simulink model "TrainingTracerVer3"  (R2025b)
settings: Solver=FixedStepAuto  StartTime=0.0  StopTime=inf  RelTol=1e-3  EnableMultiTasking=on
undefined symbols (not defined in the file): bits
libraries: stm32blockslib x11, stm32f4xxblockslib x10, svdutilitieslib x6
settings Model: STM32="{\"DigitalPortWrite\":[{\"ID\":\"Tracer_New_Version:271\"},{\"ID\":\"Tracer_New_Version:279\"},{\"ID\":\"Tracer_New_Version:277\"},{\"ID\":\"Tracer_New_Version:262\"},{\"ID\":\"TrainingTracerVer3:279\"},{\"ID\":\"TrainingTracerVer3:277\"},{\"ID\":\"TrainingTracerVer3:262\"},{\"ID\":\"TrainingTracerVer3:271\"}],\"EncoderBlock\":[{\"ID\":\"Tracer_New_Version:4\"},{\"ID\":\"Tracer_New_Version:3\"},{\"ID\":\"TrainingTracerVer3:4\"},{\"ID\":\"TrainingTracerVer3:3\"}],\"PWMOutput\":[{\"ID\":\"Tracer_New_Version:280\"},{\"ID\":\"Tracer_New_Version:278\"},{\"ID\":\"TrainingTracerVer3:280\"},{\"ID\":\"TrainingTracerVer3:278\"}],\"AnalogInput\":[{\"ID\":\"Tracer_New_Version:227\"},{\"ID\":\"Tracer_New_Version:226\"},{\"ID\":\"TrainingTracerVer3:226\"},{\"ID\":\"TrainingTracerVer3:227\"}],\"I2CControllerRead\":[{\"ID\":\"Tracer_New_Version:61\"},{\"ID\":\"Tracer_New_Version:124\"},{\"ID\":\"Tracer_New_Version:123\"},{\"ID\":\"Tracer_New_Version:187\"},{\"ID\":\"Tracer_New_Version:186\"},{\"ID\":\"Tracer_New_Version:81\"},{\"ID\":\"Tracer_New_Version:80\"},{\"ID\":\"Tracer_New_Version:144\"},{\"ID\":\"Tracer_New_Version:143\"},{\"ID\":\"Tracer_New_Version:207\"},{\"ID\":\"Tracer_New_Version:206\"},{\"ID\":\"Tracer_New_Version:103\"},{\"ID\":\"Tracer_New_Version:102\"},{\"ID\":\"Tracer_New_Version:166\"},{\"ID\":\"Tracer_New_Version:165\"},{\"ID\":\"TrainingTracerVer3:61\"},{\"ID\":\"TrainingTracerVer3:81\"},{\"ID\":\"TrainingTracerVer3:124\"},{\"ID\":\"TrainingTracerVer3:144\"},{\"ID\":\"TrainingTracerVer3:187\"},{\"ID\":\"TrainingTracerVer3:207\"}],\"DigitalPortRead\":[{\"ID\":\"Tracer_New_Version:237\"},{\"ID\":\"Tracer_New_Version:236\"},{\"ID\":\"TrainingTracerVer3:236\"},{\"ID\":\"TrainingTracerVer3:237\"}],\"I2CControllerWrite\":[{\"ID\":\"Tracer_New_Version:41\"},{\"ID\":\"Tracer_New_Version:42\"},{\"ID\":\"Tracer_New_Version:43\"},{\"ID\":\"TrainingTracerVer3:41\"},{\"ID\":\"TrainingTracerVer3:42\"},{\"ID\":\"TrainingTracerVer3:43\"}]}"  Creator=niijima  LastModifiedBy=niijima
settings OptimizationCC: EnhancedBackFolding=on  PassReuseOutputArgsAs=Individual arguments  ZeroExternalMemoryAtStartup=off  ZeroInternalMemoryAtStartup=off  MaxStackSize=512  OptimizeBlockOrder=speed  DifferentSizesBufferReuse=on  OptimizationCustomize=off  EfficientTunableParamExpr=on
settings DebuggingCC: ParameterTunabilityLossMsg=error
settings HardwareCC: ProdBitPerPointer=32.0  ProdBitPerSizeT=32.0  ProdBitPerPtrDiffT=32.0  ProdLargestAtomicInteger=Long  ProdLargestAtomicFloat=Double  ProdWordSize=32.0  ProdLongLongMode=on  ProdHWDeviceType=ARM Compatible->ARM Cortex-M
settings SFSimCC: MATLABDynamicMemAlloc=off
settings RTWCC: SystemTargetFile=ert.tlc  HardwareBoard=STM32F3xx Based  TemplateMakefile=ert_default_tmf  Toolchain=GNU Tools for ARM Embedded Processors  BuildConfiguration=Faster Runs  Description=Embedded Coder
settings CodeAppCC: ForceParamTrailComments=on  IgnoreCustomStorageClasses=off  OperatorAnnotations=on  SimulinkDataObjDesc=on  SFDataObjDesc=on  InsertBlockDesc=on
settings ERTTargetCC: ExtModeTransport=3.0  ExtModeStaticAlloc=on  ExtModeStaticAllocSize=2048.0  ExtModeMexFile=ext_xcp  ExtModeIntrfLevel=Level2 - Open  InlinedParameterPlacement=Hierarchical  DynamicArrayContainerType=coder::array  TargetLangStandard=C99 (ISO)  CodeReplacementLibrary=ARM Cortex-M  SupportContinuousTime=on

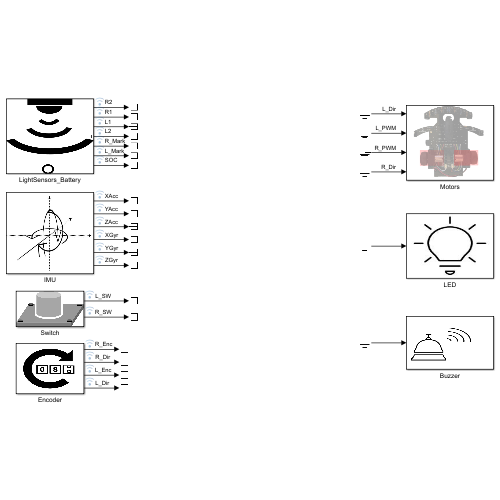
[thumbnail: Simulink's stored preview of the top-level diagram]
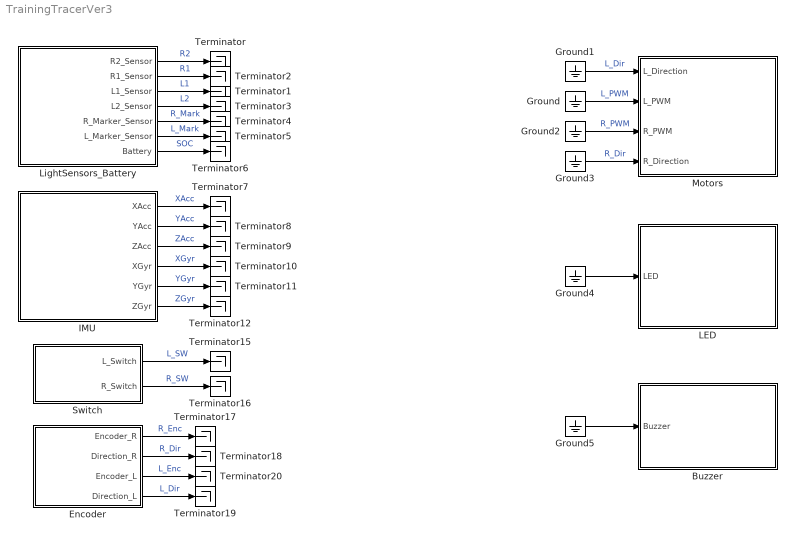
== system TrainingTracerVer3 ==
  Buzzer : Subsystem
      mask Display: image('Picture2.png');
  Encoder : Subsystem
      mask Display: image('c1d4fd0d-d243-4f64-b1ab-5e56abbdef7e.jpg');
  Ground{,1..5} (6 alike) : Ground
  IMU : Subsystem
      mask Display: image('55213469-1105-4cd9-b002-0902cf504a17.jpg');
  LED : Subsystem
      mask Display: image('c54385e9-ac3c-4890-af1e-d5685341beff.jpg');
  LightSensors_Battery : Subsystem
      mask Display: image('6109ffca-7121-49e0-b053-0876b8c7f2a6.jpg');
  Motors : Subsystem
      mask Display: image('Picture1.png');
  Switch : Subsystem
      mask Display: image('画像 (2).png');
  Terminator{,1..12,15..20} (19 alike) : Terminator
  wires:
  Encoder/2(Direction_R) -> Terminator18/1  "R_Dir"
  Encoder/1(Encoder_R) -> Terminator17/1  "R_Enc"
  Switch/2(R_Switch) -> Terminator16/1  "R_SW"
  Switch/1(L_Switch) -> Terminator15/1  "L_SW"
  IMU/6(ZGyr) -> Terminator12/1  "ZGyr"
  IMU/5(YGyr) -> Terminator11/1  "YGyr"
  IMU/4(XGyr) -> Terminator10/1  "XGyr"
  IMU/3(ZAcc) -> Terminator9/1  "ZAcc"
  IMU/2(YAcc) -> Terminator8/1  "YAcc"
  IMU/1(XAcc) -> Terminator7/1  "XAcc"
  LightSensors_Battery/7(Battery) -> Terminator6/1  "SOC"
  LightSensors_Battery/6(L_Marker_Sensor) -> Terminator5/1  "L_Mark"
  LightSensors_Battery/5(R_Marker_Sensor) -> Terminator4/1  "R_Mark"
  LightSensors_Battery/4(L2_Sensor) -> Terminator3/1  "L2"
  LightSensors_Battery/3(L1_Sensor) -> Terminator1/1  "L1"
  LightSensors_Battery/2(R1_Sensor) -> Terminator2/1  "R1"
  LightSensors_Battery/1(R2_Sensor) -> Terminator/1  "R2"
  Ground/1 -> Motors/2(L_PWM)  "L_PWM"
  Ground5/1 -> Buzzer/1(Buzzer)
  Ground4/1 -> LED/1(LED)
  Ground2/1 -> Motors/3(R_PWM)  "R_PWM"
  Ground1/1 -> Motors/1(L_Direction)  "L_Dir"
  Encoder/4(Direction_L) -> Terminator19/1  "L_Dir"
  Encoder/3(Encoder_L) -> Terminator20/1  "L_Enc"
  Ground3/1 -> Motors/4(R_Direction)  "R_Dir"

== system TrainingTracerVer3/Buzzer ==
  Buzzer : Inport
  Buzzer_ : stm32f4xxblockslib/Digital Port Write  PortName=GPIOA  PinNumber=[12]  ReadOperation=off  IOAsArray=on  EnableSimPort=off  hoistedMaskSrc=ECSoC/ECSimCodegen/Digital Port Write
      settings: LibrarySourceBlock=stm32f3xxblockslib/Digital Port Write
  wires:
  Buzzer/1 -> Buzzer_/1

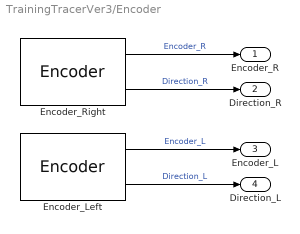
== system TrainingTracerVer3/Encoder ==
  Encoder_Left : stm32blockslib/Encoder  TimerModule=TIM1  EnableResetInput=off  OutputDirection=on  SampleTime=-1
      settings: LibrarySourceBlock=stm32f3xxblockslib/Encoder
  Encoder_Right : stm32blockslib/Encoder  TimerModule=TIM2  EnableResetInput=off  OutputDirection=on  SampleTime=-1
      settings: LibrarySourceBlock=stm32f3xxblockslib/Encoder
  Encoder_R : Outport
  Direction_R : Outport  Port=2
  Encoder_L : Outport  Port=3
  Direction_L : Outport  Port=4
  wires:
  Encoder_Right/2 -> Direction_R/1  "Direction_R"
  Encoder_Right/1 -> Encoder_R/1  "Encoder_R"
  Encoder_Left/1 -> Encoder_L/1  "Encoder_L"
  Encoder_Left/2 -> Direction_L/1  "Direction_L"

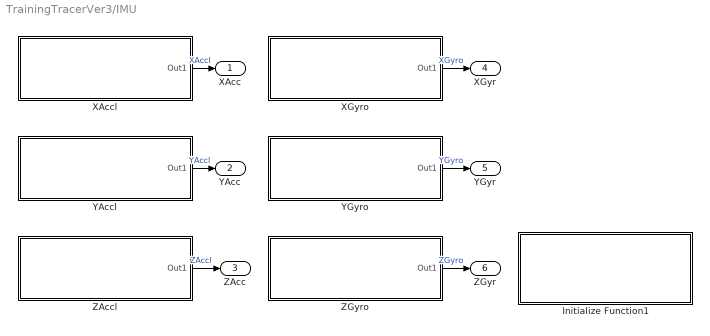
== system TrainingTracerVer3/IMU ==
  Initialize Function1 : Subsystem  TreatAsAtomicUnit=on
  XAccl : Subsystem
  XGyro : Subsystem
  YAccl : Subsystem
  YGyro : Subsystem
  ZAccl : Subsystem
  ZGyro : Subsystem
  XAcc : Outport
  YAcc : Outport  Port=2
  ZAcc : Outport  Port=3
  XGyr : Outport  Port=4
  YGyr : Outport  Port=5
  ZGyr : Outport  Port=6
  wires:
  YGyro/1(Out1) -> YGyr/1  "YGyro"
  ZGyro/1(Out1) -> ZGyr/1  "ZGyro"
  ZAccl/1(Out1) -> ZAcc/1  "ZAccl"
  XGyro/1(Out1) -> XGyr/1  "XGyro"
  YAccl/1(Out1) -> YAcc/1  "YAccl"
  XAccl/1(Out1) -> XAcc/1  "XAccl"

== system TrainingTracerVer3/LED ==
  LED : Inport
  LED_ : stm32f4xxblockslib/Digital Port Write  PortName=GPIOB  PinNumber=[3]  ReadOperation=off  IOAsArray=on  EnableSimPort=off  hoistedMaskSrc=ECSoC/ECSimCodegen/Digital Port Write
      settings: LibrarySourceBlock=stm32f3xxblockslib/Digital Port Write
  wires:
  LED/1 -> LED_/1

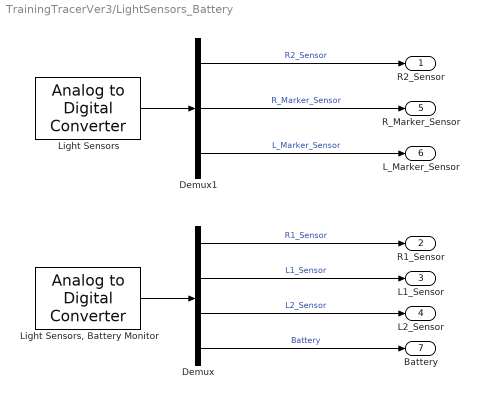
== system TrainingTracerVer3/LightSensors_Battery ==
  Demux : Demux
  Demux1 : Demux  Outputs=3
  Light Sensors : stm32f4xxblockslib/Analog to Digital Converter  ADCModule=ADC1  ConversionGroup=Regular  TriggerMode=Trigger and read  NumberOfConversions=3  EnableBufferConv=off  BufferLength=1  OutputStatus=off  SampleTime=-1  EnableSimPort=off  hoistedMaskSrc=ECSoC/ECSimCodegen/Analog to Digital Converter
      settings: LibrarySourceBlock=stm32f3xxblockslib/Analog to Digital Converter
  "Light Sensors, Battery Monitor" : stm32f4xxblockslib/Analog to Digital Converter  ADCModule=ADC2  ConversionGroup=Regular  TriggerMode=Trigger and read  NumberOfConversions=4  EnableBufferConv=off  BufferLength=1  OutputStatus=off  SampleTime=-1  EnableSimPort=off  hoistedMaskSrc=ECSoC/ECSimCodegen/Analog to Digital Converter
      settings: LibrarySourceBlock=stm32f3xxblockslib/Analog to Digital Converter
  R2_Sensor : Outport
  R1_Sensor : Outport  Port=2
  L1_Sensor : Outport  Port=3
  L2_Sensor : Outport  Port=4
  R_Marker_Sensor : Outport  Port=5
  L_Marker_Sensor : Outport  Port=6
  Battery : Outport  Port=7
  wires:
  Demux/2 -> L1_Sensor/1  "L1_Sensor"
  "Light Sensors, Battery Monitor"/1 -> Demux/1
  Demux1/1 -> R2_Sensor/1  "R2_Sensor"
  Light Sensors/1 -> Demux1/1
  Demux/3 -> L2_Sensor/1  "L2_Sensor"
  Demux1/3 -> L_Marker_Sensor/1  "L_Marker_Sensor"
  Demux1/2 -> R_Marker_Sensor/1  "R_Marker_Sensor"
  Demux/4 -> Battery/1  "Battery"
  Demux/1 -> R1_Sensor/1  "R1_Sensor"

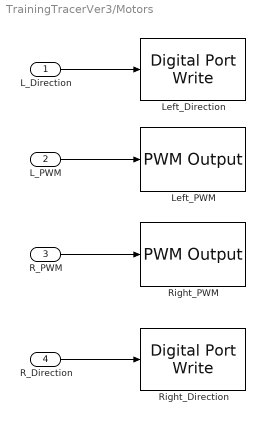
== system TrainingTracerVer3/Motors ==
  L_Direction : Inport
  L_PWM : Inport  Port=2
  R_PWM : Inport  Port=3
  R_Direction : Inport  Port=4
  Left_Direction : stm32f4xxblockslib/Digital Port Write  PortName=GPIOA  PinNumber=[10]  ReadOperation=off  IOAsArray=on  EnableSimPort=off  hoistedMaskSrc=ECSoC/ECSimCodegen/Digital Port Write
      settings: LibrarySourceBlock=stm32f3xxblockslib/Digital Port Write
  Left_PWM : stm32f4xxblockslib/PWM Output  ProcessorFamily=STM32F3  TimerModule=TIM16  DutycycleUnits=Percentage  EnableChannel1=on  EnableCaptureCompare1Input=off  EnableCaptureCompare1ComplementaryInput=off  EnableOutputCompare1ModeInput=off  EnableChannel2=off  EnableCaptureCompare2Input=off  EnableCaptureCompare2ComplementaryInput=off  EnableOutputCompare2ModeInput=off  EnableChannel3=off  EnableCaptureCompare3Input=off  EnableCaptureCompare3ComplementaryInput=off  EnableOutputCompare3ModeInput=off  EnableChannel4=on  EnableCaptureCompare4Input=off  EnableCaptureCompare4ComplementaryInput=off  EnableOutputCompare4ModeInput=off  EnableChannel5=off  EnableCaptureCompare5Input=off  EnableOutputCompare5ModeInput=off  EnableChannel6=off  EnableCaptureCompare6Input=off  EnableOutputCompare6ModeInput=off  EnableCounterInput=off  EnableMainOutputInput=off  EnableFrequencyInput=off  SetRCAfterCE=off  OutputDirection=off  OutputMainOutputEnableStatus=off  SampleTime=0.1  EnableSimPort=off  EnableUpdateEvent=off  EnableCaptureCompare1Event=off  EnableCaptureCompare2Event=off  EnableCaptureCompare3Event=off  EnableCaptureCompare4Event=off  EnableTriggerEvent=off  EnableBreakEvent=off  EnableBreakEvent2=off  hoistedMaskSrc=ECSoC/ECSimCodegen/PWM Output
      settings: LibrarySourceBlock=stm32f3xxblockslib/PWM Output
  Right_Direction : stm32f4xxblockslib/Digital Port Write  PortName=GPIOA  PinNumber=[11]  ReadOperation=off  IOAsArray=on  EnableSimPort=off  hoistedMaskSrc=ECSoC/ECSimCodegen/Digital Port Write
      settings: LibrarySourceBlock=stm32f3xxblockslib/Digital Port Write
  Right_PWM : stm32f4xxblockslib/PWM Output  ProcessorFamily=STM32F3  TimerModule=TIM17  DutycycleUnits=Percentage  EnableChannel1=on  EnableCaptureCompare1Input=off  EnableCaptureCompare1ComplementaryInput=off  EnableOutputCompare1ModeInput=off  EnableChannel2=off  EnableCaptureCompare2Input=off  EnableCaptureCompare2ComplementaryInput=off  EnableOutputCompare2ModeInput=off  EnableChannel3=off  EnableCaptureCompare3Input=off  EnableCaptureCompare3ComplementaryInput=off  EnableOutputCompare3ModeInput=off  EnableChannel4=off  EnableCaptureCompare4Input=off  EnableCaptureCompare4ComplementaryInput=off  EnableOutputCompare4ModeInput=off  EnableChannel5=off  EnableCaptureCompare5Input=off  EnableOutputCompare5ModeInput=off  EnableChannel6=off  EnableCaptureCompare6Input=off  EnableOutputCompare6ModeInput=off  EnableCounterInput=off  EnableMainOutputInput=off  EnableFrequencyInput=off  SetRCAfterCE=off  OutputDirection=off  OutputMainOutputEnableStatus=off  SampleTime=0.1  EnableSimPort=off  EnableUpdateEvent=off  EnableCaptureCompare1Event=off  EnableCaptureCompare2Event=off  EnableCaptureCompare3Event=off  EnableCaptureCompare4Event=off  EnableTriggerEvent=off  EnableBreakEvent=off  EnableBreakEvent2=off  hoistedMaskSrc=ECSoC/ECSimCodegen/PWM Output
      settings: LibrarySourceBlock=stm32f3xxblockslib/PWM Output
  wires:
  R_Direction/1 -> Right_Direction/1
  R_PWM/1 -> Right_PWM/1
  L_Direction/1 -> Left_Direction/1
  L_PWM/1 -> Left_PWM/1

== system TrainingTracerVer3/Switch ==
  L_Switch_ : stm32f4xxblockslib/Digital Port Read  PortName=GPIOF  PinNumber=[0]  ReadOperation=on  IOAsArray=off  SampleTime=-1  EnableSimPort=off  hoistedMaskSrc=ECSoC/ECSimCodegen/Digital Port Read
      settings: LibrarySourceBlock=stm32f3xxblockslib/Digital Port Read
  R_Switch_ : stm32f4xxblockslib/Digital Port Read  PortName=GPIOF  PinNumber=[1]  ReadOperation=on  IOAsArray=off  SampleTime=-1  EnableSimPort=off  hoistedMaskSrc=ECSoC/ECSimCodegen/Digital Port Read
      settings: LibrarySourceBlock=stm32f3xxblockslib/Digital Port Read
  L_Switch : Outport
  R_Switch : Outport  Port=2
  wires:
  R_Switch_/1 -> R_Switch/1  "R_Switch"
  L_Switch_/1 -> L_Switch/1  "L_Switch"

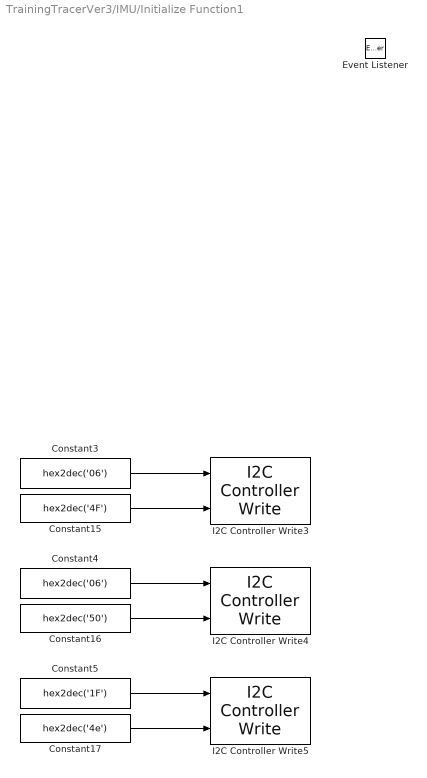
== system TrainingTracerVer3/IMU/Initialize Function1 ==
  Constant15 : Constant  Value=hex2dec('4F')  OutDataTypeStr=uint8
  Constant16 : Constant  Value=hex2dec('50')  OutDataTypeStr=uint8
  Constant17 : Constant  Value=hex2dec('4e')  OutDataTypeStr=uint8
  Constant3 : Constant  Value=hex2dec('06')  VectorParams1D=off  OutDataTypeStr=uint8
  Constant4 : Constant  Value=hex2dec('06')  VectorParams1D=off  OutDataTypeStr=uint8
  Constant5 : Constant  Value=hex2dec('1F')  VectorParams1D=off  OutDataTypeStr=uint8
  Event Listener : EventListener  DisableCoverage=on  EventName=reset
  I2C Controller Write3 : stm32blockslib/I2C Controller Write  I2CModule=I2C1  Mode=Controller  AddressingMode=7-bits  PeripheralByteOrder=LittleEndian  OwnPeripheralAddress=uint8(170)  PeripheralAddressVia=Dialog  PeripheralAddress=hex2dec('69')  RegisterAddressMode=on  RegisterAddressVia=Inport  RegisterAddress=hex2dec('0F')  RepeatedStart=off  NoAck=off  OutputStatus=off  BlockMode=Transmit  DataType=uint8  DataLength=1  Timeout=0.1  SampleTime=-1
      settings: LibrarySourceBlock=stm32f4xxblockslib/I2C Controller Write
  I2C Controller Write4 : stm32blockslib/I2C Controller Write  I2CModule=I2C1  Mode=Controller  AddressingMode=7-bits  PeripheralByteOrder=LittleEndian  OwnPeripheralAddress=uint8(170)  PeripheralAddressVia=Dialog  PeripheralAddress=hex2dec('69')  RegisterAddressMode=on  RegisterAddressVia=Inport  RegisterAddress=hex2dec('10')  RepeatedStart=off  NoAck=off  OutputStatus=off  BlockMode=Transmit  DataType=uint8  DataLength=1  Timeout=0.1  SampleTime=-1
      settings: LibrarySourceBlock=stm32f4xxblockslib/I2C Controller Write
  I2C Controller Write5 : stm32blockslib/I2C Controller Write  I2CModule=I2C1  Mode=Controller  AddressingMode=7-bits  PeripheralByteOrder=LittleEndian  OwnPeripheralAddress=uint8(170)  PeripheralAddressVia=Dialog  PeripheralAddress=hex2dec('69')  RegisterAddressMode=on  RegisterAddressVia=Inport  RegisterAddress=hex2dec('11')  RepeatedStart=off  NoAck=off  OutputStatus=off  BlockMode=Transmit  DataType=uint8  DataLength=1  Timeout=0.1  SampleTime=-1
      settings: LibrarySourceBlock=stm32f4xxblockslib/I2C Controller Write
  wires:
  Constant5/1 -> I2C Controller Write5/1
  Constant4/1 -> I2C Controller Write4/1
  Constant3/1 -> I2C Controller Write3/1
  Constant15/1 -> I2C Controller Write3/2
  Constant16/1 -> I2C Controller Write4/2
  Constant17/1 -> I2C Controller Write5/2

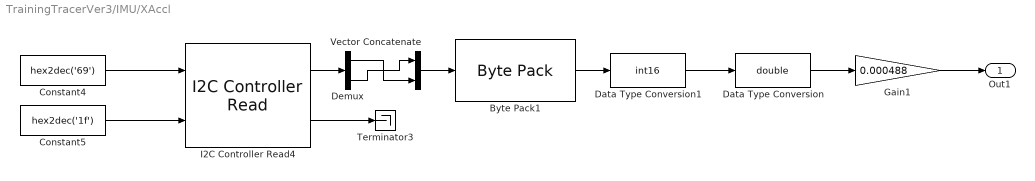
== system TrainingTracerVer3/IMU/XAccl ==
  Byte Pack1 : svdutilitieslib/Byte Pack  maskPackedDataType=uint16  datatypes={'uint8'}  byteAlign=1  blockPlatform=arduinoert
      settings: LibrarySourceBlock=mcblib/Signal Management/Byte Pack
  Constant4 : Constant  Value=hex2dec('69')  OutDataTypeStr=uint8
  Constant5 : Constant  Value=hex2dec('1f')  OutDataTypeStr=uint8
  Data Type Conversion : DataTypeConversion  OutDataTypeStr=double  SaturateOnIntegerOverflow=off  RndMeth=Floor
  Data Type Conversion1 : DataTypeConversion  OutDataTypeStr=int16  SaturateOnIntegerOverflow=off  RndMeth=Floor
  Demux : Demux  Outputs=2
  Gain1 : Gain  Gain=0.000488
  I2C Controller Read4 : stm32blockslib/I2C Controller Read  I2CModule=I2C1  Mode=Controller  AddressingMode=7-bits  PeripheralByteOrder=BigEndian  OwnPeripheralAddress=uint8(170)  PeripheralAddressVia=Inport  PeripheralAddress=0x19  RegisterAddressMode=on  RegisterAddressVia=Inport  RegisterAddress=0x02  RepeatedStart=off  NoAck=off  OutputStatus=on  BlockMode=Receive  DataType=uint8  DataLength=2  Timeout=0.1  SampleTime=-1
      settings: LibrarySourceBlock=stm32f4xxblockslib/I2C Controller Read
  Terminator3 : Terminator
  Vector Concatenate : Concatenate
  Out1 : Outport
  wires:
  Constant4/1 -> I2C Controller Read4/1
  I2C Controller Read4/2 -> Terminator3/1
  Constant5/1 -> I2C Controller Read4/2
  Byte Pack1/1 -> Data Type Conversion1/1
  Vector Concatenate/1 -> Byte Pack1/1
  Demux/1 -> Vector Concatenate/2
  Demux/2 -> Vector Concatenate/1
  I2C Controller Read4/1 -> Demux/1
  Data Type Conversion1/1 -> Data Type Conversion/1
  Gain1/1 -> Out1/1
  Data Type Conversion/1 -> Gain1/1

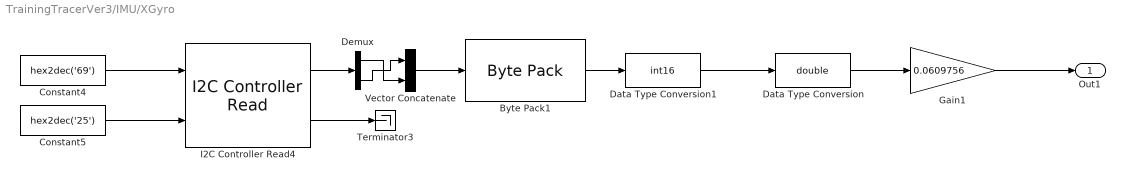
== system TrainingTracerVer3/IMU/XGyro ==
  Byte Pack1 : svdutilitieslib/Byte Pack  maskPackedDataType=uint16  datatypes={'uint8'}  byteAlign=1  blockPlatform=arduinoert
      settings: LibrarySourceBlock=mcblib/Signal Management/Byte Pack
  Constant4 : Constant  Value=hex2dec('69')  OutDataTypeStr=uint8
  Constant5 : Constant  Value=hex2dec('25')  OutDataTypeStr=uint8
  Data Type Conversion : DataTypeConversion  OutDataTypeStr=double  SaturateOnIntegerOverflow=off  RndMeth=Floor
  Data Type Conversion1 : DataTypeConversion  OutDataTypeStr=int16  SaturateOnIntegerOverflow=off  RndMeth=Floor
  Demux : Demux  Outputs=2
  Gain1 : Gain  Gain=0.0609756
  I2C Controller Read4 : stm32blockslib/I2C Controller Read  I2CModule=I2C1  Mode=Controller  AddressingMode=7-bits  PeripheralByteOrder=BigEndian  OwnPeripheralAddress=uint8(170)  PeripheralAddressVia=Inport  PeripheralAddress=0x19  RegisterAddressMode=on  RegisterAddressVia=Inport  RegisterAddress=0x02  RepeatedStart=off  NoAck=off  OutputStatus=on  BlockMode=Receive  DataType=uint8  DataLength=2  Timeout=0.1  SampleTime=-1
      settings: LibrarySourceBlock=stm32f4xxblockslib/I2C Controller Read
  Terminator3 : Terminator
  Vector Concatenate : Concatenate
  Out1 : Outport
  wires:
  Constant4/1 -> I2C Controller Read4/1
  I2C Controller Read4/2 -> Terminator3/1
  Constant5/1 -> I2C Controller Read4/2
  Vector Concatenate/1 -> Byte Pack1/1
  Gain1/1 -> Out1/1
  Data Type Conversion1/1 -> Data Type Conversion/1
  Byte Pack1/1 -> Data Type Conversion1/1
  I2C Controller Read4/1 -> Demux/1
  Demux/1 -> Vector Concatenate/2
  Demux/2 -> Vector Concatenate/1
  Data Type Conversion/1 -> Gain1/1

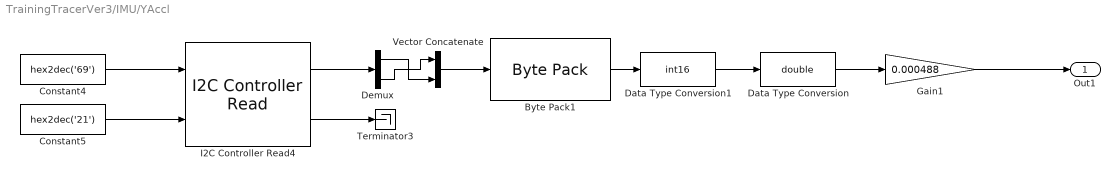
== system TrainingTracerVer3/IMU/YAccl ==
  Byte Pack1 : svdutilitieslib/Byte Pack  maskPackedDataType=uint16  datatypes={'uint8'}  byteAlign=1  blockPlatform=arduinoert
      settings: LibrarySourceBlock=mcblib/Signal Management/Byte Pack
  Constant4 : Constant  Value=hex2dec('69')  OutDataTypeStr=uint8
  Constant5 : Constant  Value=hex2dec('21')  OutDataTypeStr=uint8
  Data Type Conversion : DataTypeConversion  OutDataTypeStr=double  SaturateOnIntegerOverflow=off  RndMeth=Floor
  Data Type Conversion1 : DataTypeConversion  OutDataTypeStr=int16  SaturateOnIntegerOverflow=off  RndMeth=Floor
  Demux : Demux  Outputs=2
  Gain1 : Gain  Gain=0.000488
  I2C Controller Read4 : stm32blockslib/I2C Controller Read  I2CModule=I2C1  Mode=Controller  AddressingMode=7-bits  PeripheralByteOrder=BigEndian  OwnPeripheralAddress=uint8(170)  PeripheralAddressVia=Inport  PeripheralAddress=0x19  RegisterAddressMode=on  RegisterAddressVia=Inport  RegisterAddress=0x02  RepeatedStart=off  NoAck=off  OutputStatus=on  BlockMode=Receive  DataType=uint8  DataLength=2  Timeout=0.1  SampleTime=-1
      settings: LibrarySourceBlock=stm32f4xxblockslib/I2C Controller Read
  Terminator3 : Terminator
  Vector Concatenate : Concatenate
  Out1 : Outport
  wires:
  Constant4/1 -> I2C Controller Read4/1
  I2C Controller Read4/2 -> Terminator3/1
  Constant5/1 -> I2C Controller Read4/2
  Vector Concatenate/1 -> Byte Pack1/1
  Byte Pack1/1 -> Data Type Conversion1/1
  Data Type Conversion1/1 -> Data Type Conversion/1
  I2C Controller Read4/1 -> Demux/1
  Demux/2 -> Vector Concatenate/1
  Demux/1 -> Vector Concatenate/2
  Gain1/1 -> Out1/1
  Data Type Conversion/1 -> Gain1/1

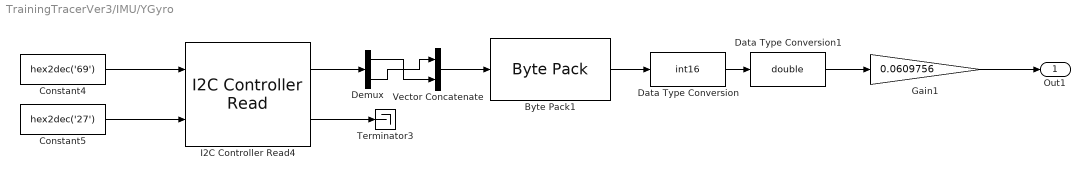
== system TrainingTracerVer3/IMU/YGyro ==
  Byte Pack1 : svdutilitieslib/Byte Pack  maskPackedDataType=uint16  datatypes={'uint8'}  byteAlign=1  blockPlatform=arduinoert
      settings: LibrarySourceBlock=mcblib/Signal Management/Byte Pack
  Constant4 : Constant  Value=hex2dec('69')  OutDataTypeStr=uint8
  Constant5 : Constant  Value=hex2dec('27')  OutDataTypeStr=uint8
  Data Type Conversion : DataTypeConversion  OutDataTypeStr=int16  SaturateOnIntegerOverflow=off  RndMeth=Floor
  Data Type Conversion1 : DataTypeConversion  OutDataTypeStr=double  SaturateOnIntegerOverflow=off  RndMeth=Floor
  Demux : Demux  Outputs=2
  Gain1 : Gain  Gain=0.0609756
  I2C Controller Read4 : stm32blockslib/I2C Controller Read  I2CModule=I2C1  Mode=Controller  AddressingMode=7-bits  PeripheralByteOrder=BigEndian  OwnPeripheralAddress=uint8(170)  PeripheralAddressVia=Inport  PeripheralAddress=0x19  RegisterAddressMode=on  RegisterAddressVia=Inport  RegisterAddress=0x02  RepeatedStart=off  NoAck=off  OutputStatus=on  BlockMode=Receive  DataType=uint8  DataLength=2  Timeout=0.1  SampleTime=-1
      settings: LibrarySourceBlock=stm32f4xxblockslib/I2C Controller Read
  Terminator3 : Terminator
  Vector Concatenate : Concatenate
  Out1 : Outport
  wires:
  Constant4/1 -> I2C Controller Read4/1
  I2C Controller Read4/2 -> Terminator3/1
  Constant5/1 -> I2C Controller Read4/2
  Vector Concatenate/1 -> Byte Pack1/1
  I2C Controller Read4/1 -> Demux/1
  Demux/2 -> Vector Concatenate/1
  Demux/1 -> Vector Concatenate/2
  Byte Pack1/1 -> Data Type Conversion/1
  Data Type Conversion/1 -> Data Type Conversion1/1
  Gain1/1 -> Out1/1
  Data Type Conversion1/1 -> Gain1/1

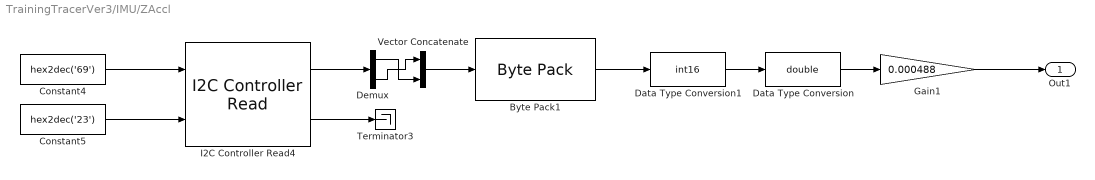
== system TrainingTracerVer3/IMU/ZAccl ==
  Byte Pack1 : svdutilitieslib/Byte Pack  maskPackedDataType=uint16  datatypes={'uint8'}  byteAlign=1  blockPlatform=arduinoert
      settings: LibrarySourceBlock=mcblib/Signal Management/Byte Pack
  Constant4 : Constant  Value=hex2dec('69')  OutDataTypeStr=uint8
  Constant5 : Constant  Value=hex2dec('23')  OutDataTypeStr=uint8
  Data Type Conversion : DataTypeConversion  OutDataTypeStr=double  SaturateOnIntegerOverflow=off  RndMeth=Floor
  Data Type Conversion1 : DataTypeConversion  OutDataTypeStr=int16  SaturateOnIntegerOverflow=off  RndMeth=Floor
  Demux : Demux  Outputs=2
  Gain1 : Gain  Gain=0.000488
  I2C Controller Read4 : stm32blockslib/I2C Controller Read  I2CModule=I2C1  Mode=Controller  AddressingMode=7-bits  PeripheralByteOrder=BigEndian  OwnPeripheralAddress=uint8(170)  PeripheralAddressVia=Inport  PeripheralAddress=0x19  RegisterAddressMode=on  RegisterAddressVia=Inport  RegisterAddress=0x02  RepeatedStart=off  NoAck=off  OutputStatus=on  BlockMode=Receive  DataType=uint8  DataLength=2  Timeout=0.1  SampleTime=-1
      settings: LibrarySourceBlock=stm32f4xxblockslib/I2C Controller Read
  Terminator3 : Terminator
  Vector Concatenate : Concatenate
  Out1 : Outport
  wires:
  Constant4/1 -> I2C Controller Read4/1
  I2C Controller Read4/2 -> Terminator3/1
  Constant5/1 -> I2C Controller Read4/2
  Vector Concatenate/1 -> Byte Pack1/1
  I2C Controller Read4/1 -> Demux/1
  Demux/1 -> Vector Concatenate/2
  Demux/2 -> Vector Concatenate/1
  Byte Pack1/1 -> Data Type Conversion1/1
  Data Type Conversion1/1 -> Data Type Conversion/1
  Gain1/1 -> Out1/1
  Data Type Conversion/1 -> Gain1/1

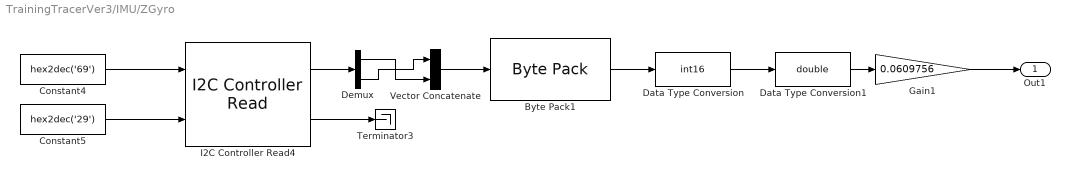
== system TrainingTracerVer3/IMU/ZGyro ==
  Byte Pack1 : svdutilitieslib/Byte Pack  maskPackedDataType=uint16  datatypes={'uint8'}  byteAlign=1  blockPlatform=arduinoert
      settings: LibrarySourceBlock=mcblib/Signal Management/Byte Pack
  Constant4 : Constant  Value=hex2dec('69')  OutDataTypeStr=uint8
  Constant5 : Constant  Value=hex2dec('29')  OutDataTypeStr=uint8
  Data Type Conversion : DataTypeConversion  OutDataTypeStr=int16  SaturateOnIntegerOverflow=off  RndMeth=Floor
  Data Type Conversion1 : DataTypeConversion  OutDataTypeStr=double  SaturateOnIntegerOverflow=off  RndMeth=Floor
  Demux : Demux  Outputs=2
  Gain1 : Gain  Gain=0.0609756
  I2C Controller Read4 : stm32blockslib/I2C Controller Read  I2CModule=I2C1  Mode=Controller  AddressingMode=7-bits  PeripheralByteOrder=BigEndian  OwnPeripheralAddress=uint8(170)  PeripheralAddressVia=Inport  PeripheralAddress=0x19  RegisterAddressMode=on  RegisterAddressVia=Inport  RegisterAddress=0x02  RepeatedStart=off  NoAck=off  OutputStatus=on  BlockMode=Receive  DataType=uint8  DataLength=2  Timeout=0.001  SampleTime=-1
      settings: LibrarySourceBlock=stm32f4xxblockslib/I2C Controller Read
  Terminator3 : Terminator
  Vector Concatenate : Concatenate
  Out1 : Outport
  wires:
  Constant4/1 -> I2C Controller Read4/1
  I2C Controller Read4/2 -> Terminator3/1
  Constant5/1 -> I2C Controller Read4/2
  Vector Concatenate/1 -> Byte Pack1/1
  I2C Controller Read4/1 -> Demux/1
  Demux/2 -> Vector Concatenate/1
  Demux/1 -> Vector Concatenate/2
  Byte Pack1/1 -> Data Type Conversion/1
  Data Type Conversion/1 -> Data Type Conversion1/1
  Gain1/1 -> Out1/1
  Data Type Conversion1/1 -> Gain1/1
